simulink model "single_camera_xy_tracking_base_cv_kf_pre_fix"  (R2025b)
settings: Solver=FixedStepDiscrete  StartTime=0  StopTime=T_end  FixedStep=Ts  RelTol=1e-3
InitFcn:
  | config_dir=fullfile(fileparts(get_param(bdroot,'FileName')),'..','config');
  | addpath(config_dir);
  | init_single_camera_xy_tracking_base_cv_kf;
values from neighbouring files (symbols this model uses):
  Kpx = parameters(3)    [build_single_camera_joint_velocity_direct.m]    (also in build_single_camera_joint_velocity_direct1.m)
  Kpy = parameters(4);",  "k_ff=parameters(5)    [build_single_camera_joint_velocity_direct.m]    (also in build_single_camera_joint_velocity_direct1.m)
  Z_hat = parameters(2)    [build_single_camera_joint_velocity_direct.m]    (also in build_single_camera_joint_velocity_direct1.m)
undefined symbols (not defined in the file or in its folder): a_xy_max, controller_enable, data, data_SL_Info, ekf_reset_timeout_sec, enable_ekf_feedforward, enable_proportional, ff_ramp_time, joint_state_timeout_sec, k_ff, measurement_reset_timeout, nis_position_threshold, nis_velocity_threshold, P0, Q_kf, R_position, R_velocity, required_valid_frames, target_timeout_sec, Ts, v_xy_max
libraries: ros2lib x5, robotmaniplib x2
Description:
  | Base-frame four-state CV Kalman Filter. Python velocity is camera-frame relative velocity; measured camera twist is compensated before KF updates.
settings Model: Creator=ASUS  LastModifiedBy=ASUS
settings DataIOCC: SignalLogging=off

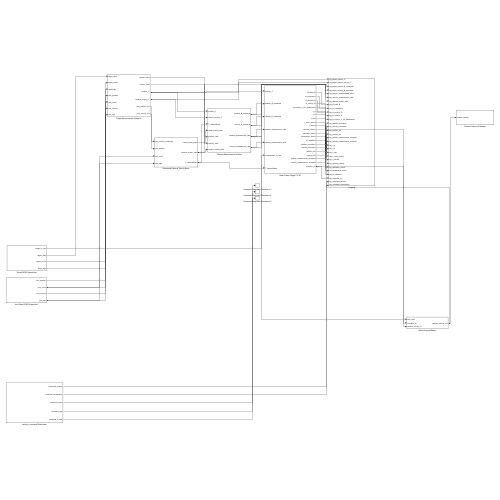
[thumbnail: Simulink's stored preview of the top-level diagram]
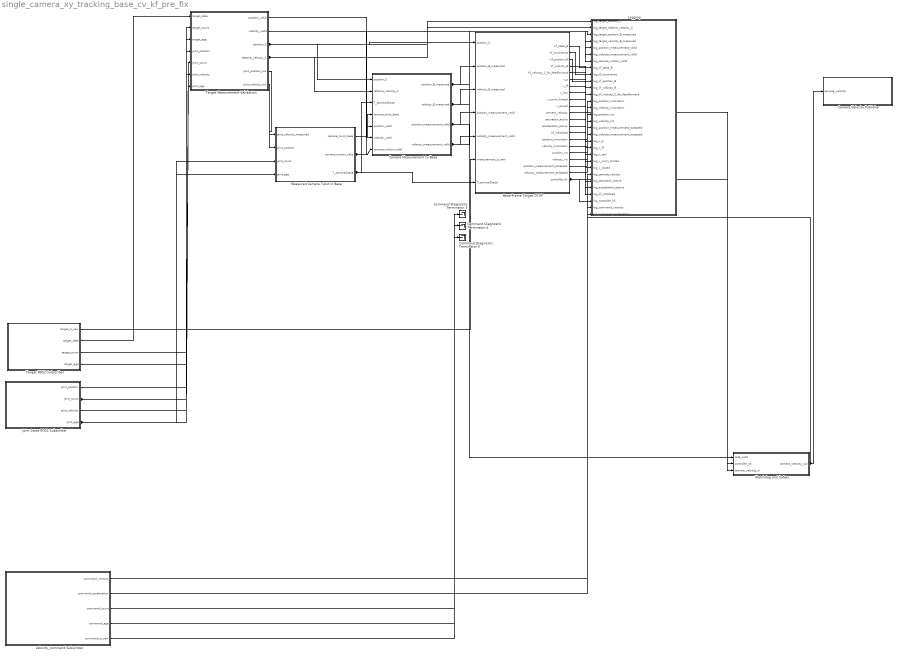
== system single_camera_xy_tracking_base_cv_kf_pre_fix ==
  Base-Frame Target CV KF : Subsystem
  Camera Measurement to Base : Subsystem
  Camera Velocity Publisher : Subsystem
  Command Diagnostic Terminator 3 : Terminator
  Command Diagnostic Terminator 4 : Terminator
  Command Diagnostic Terminator 5 : Terminator
  Joint State ROS2 Subscriber : Subsystem
  Logging : Subsystem
  Measured Camera Twist in Base : Subsystem
  Target Measurement Validation : Subsystem
  Target ROS2 Subscriber : Subsystem
  Watchdog and Safety : Subsystem
  velocity_command Subscriber : Subsystem
  wires:
  Target ROS2 Subscriber/2(target_data) -> Target Measurement Validation/1(target_data)
  Target ROS2 Subscriber/3(target_count) -> Target Measurement Validation/2(target_count)
  Target ROS2 Subscriber/4(target_age) -> Target Measurement Validation/3(target_age)
  Joint State ROS2 Subscriber/1(joint_position) -> Target Measurement Validation/4(joint_position)
  Joint State ROS2 Subscriber/2(joint_count) -> Target Measurement Validation/5(joint_count), Measured Camera Twist in Base/3(joint_count)
  Joint State ROS2 Subscriber/3(joint_velocity) -> Target Measurement Validation/6(joint_velocity)
  Joint State ROS2 Subscriber/4(joint_age) -> Target Measurement Validation/7(joint_age), Measured Camera Twist in Base/4(joint_age)
  Target Measurement Validation/6(joint_velocity_out) -> Measured Camera Twist in Base/1(joint_velocity_measured)
  Target Measurement Validation/5(joint_position_out) -> Measured Camera Twist in Base/2(joint_position)
  Target Measurement Validation/3(position_C) -> Camera Measurement to Base/1(position_C), Base-Frame Target CV KF/1(position_C), Logging/1(log_target_position_C)
  Target Measurement Validation/4(relative_velocity_C) -> Camera Measurement to Base/2(relative_velocity_C), Logging/2(log_target_relative_velocity_C)
  Measured Camera Twist in Base/3(T_camera2base) -> Camera Measurement to Base/3(T_camera2base), Base-Frame Target CV KF/7(T_camera2base)
  Measured Camera Twist in Base/1(camera_twist_base) -> Camera Measurement to Base/4(camera_twist_base)
  Target Measurement Validation/1(position_valid) -> Camera Measurement to Base/5(position_valid)
  Target Measurement Validation/2(velocity_valid) -> Camera Measurement to Base/6(velocity_valid)
  Measured Camera Twist in Base/2(camera_motion_valid) -> Camera Measurement to Base/7(camera_motion_valid), Logging/7(log_camera_motion_valid)
  Camera Measurement to Base/1(position_B_measured) -> Base-Frame Target CV KF/2(position_B_measured), Logging/3(log_target_position_B_measured)
  Camera Measurement to Base/2(velocity_B_measured) -> Base-Frame Target CV KF/3(velocity_B_measured), Logging/4(log_target_velocity_B_measured)
  Camera Measurement to Base/3(position_measurement_valid) -> Base-Frame Target CV KF/4(position_measurement_valid), Watchdog and Safety/1(safe_valid), Logging/5(log_position_measurement_valid)
  Camera Measurement to Base/4(velocity_measurement_valid) -> Base-Frame Target CV KF/5(velocity_measurement_valid), Logging/6(log_velocity_measurement_valid)
  Target ROS2 Subscriber/1(target_is_new) -> Base-Frame Target CV KF/6(measurement_is_new)
  Base-Frame Target CV KF/21(controller_ok) -> Watchdog and Safety/2(controller_ok), Logging/28(log_controller_ok)
  Base-Frame Target CV KF/11(camera_velocity) -> Watchdog and Safety/3(camera_velocity_in)
  Watchdog and Safety/1(camera_velocity_out) -> Camera Velocity Publisher/1(camera_velocity), Logging/24(log_camera_velocity)
  Base-Frame Target CV KF/1(kf_state_B) -> Logging/8(log_kf_state_B)
  Base-Frame Target CV KF/2(kf_covariance) -> Logging/9(log_kf_covariance)
  Base-Frame Target CV KF/3(kf_position_B) -> Logging/10(log_kf_position_B)
  Base-Frame Target CV KF/4(kf_velocity_B) -> Logging/11(log_kf_velocity_B)
  Base-Frame Target CV KF/5(kf_velocity_C_for_feedforward) -> Logging/12(log_kf_velocity_C_for_feedforward)
  Base-Frame Target CV KF/15(position_innovation) -> Logging/13(log_position_innovation)
  Base-Frame Target CV KF/16(velocity_innovation) -> Logging/14(log_velocity_innovation)
  Base-Frame Target CV KF/17(position_nis) -> Logging/15(log_position_nis)
  Base-Frame Target CV KF/18(velocity_nis) -> Logging/16(log_velocity_nis)
  Base-Frame Target CV KF/19(position_measurement_accepted) -> Logging/17(log_position_measurement_accepted)
  Base-Frame Target CV KF/20(velocity_measurement_accepted) -> Logging/18(log_velocity_measurement_accepted)
  Base-Frame Target CV KF/6(v_p) -> Logging/19(log_v_p)
  Base-Frame Target CV KF/7(v_ff) -> Logging/20(log_v_ff)
  Base-Frame Target CV KF/8(v_raw) -> Logging/21(log_v_raw)
  Base-Frame Target CV KF/9(v_norm_limited) -> Logging/22(log_v_norm_limited)
  Base-Frame Target CV KF/10(v_issued) -> Logging/23(log_v_issued)
  Base-Frame Target CV KF/12(saturation_active) -> Logging/25(log_saturation_active)
  Base-Frame Target CV KF/13(acceleration_active) -> Logging/26(log_acceleration_active)
  Base-Frame Target CV KF/14(kf_initialized) -> Logging/27(log_kf_initialized)
  velocity_command Subscriber/1(command_velocity) -> Logging/29(log_command_velocity)
  velocity_command Subscriber/2(command_acceleration) -> Logging/30(log_command_acceleration)
  velocity_command Subscriber/3(command_count) -> Command Diagnostic Terminator 3/1
  velocity_command Subscriber/4(command_age) -> Command Diagnostic Terminator 4/1
  velocity_command Subscriber/5(command_is_new) -> Command Diagnostic Terminator 5/1

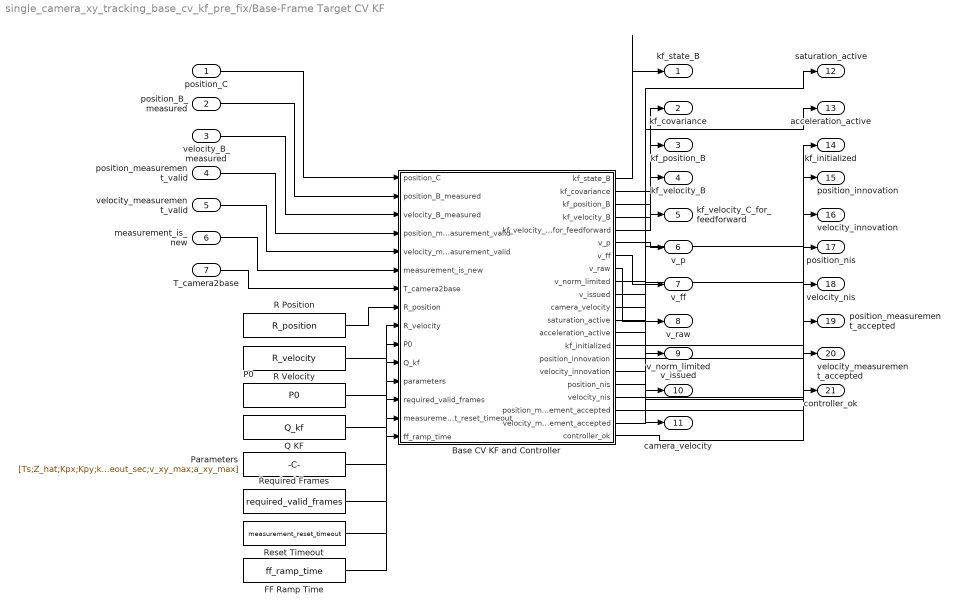
== system single_camera_xy_tracking_base_cv_kf_pre_fix/Base-Frame Target CV KF ==
  position_C : Inport
  position_B_measured : Inport  Port=2
  velocity_B_measured : Inport  Port=3
  position_measurement_valid : Inport  Port=4
  velocity_measurement_valid : Inport  Port=5
  measurement_is_new : Inport  Port=6
  T_camera2base : Inport  Port=7
  Base CV KF and Controller : MATLAB Function  TreatAsAtomicUnit=on
  FF Ramp Time : Constant  Value=ff_ramp_time
  P0 : Constant  Value=P0
  Parameters : Constant  Value=[Ts;Z_hat;Kpx;Kpy;k_ff;nis_position_threshold;nis_velocity_threshold;double(enable_proportional);double(enable_ekf_feedforward);double(controller_enable);ekf_reset_timeout_sec;v_xy_max;a_xy_max]
  Q KF : Constant  Value=Q_kf
  R Position : Constant  Value=R_position
  R Velocity : Constant  Value=R_velocity
  Required Frames : Constant  Value=required_valid_frames
  Reset Timeout : Constant  Value=measurement_reset_timeout
  kf_state_B : Outport
  kf_covariance : Outport  Port=2
  kf_position_B : Outport  Port=3
  kf_velocity_B : Outport  Port=4
  kf_velocity_C_for_feedforward : Outport  Port=5
  v_p : Outport  Port=6
  v_ff : Outport  Port=7
  v_raw : Outport  Port=8
  v_norm_limited : Outport  Port=9
  v_issued : Outport  Port=10
  camera_velocity : Outport  Port=11
  saturation_active : Outport  Port=12
  acceleration_active : Outport  Port=13
  kf_initialized : Outport  Port=14
  position_innovation : Outport  Port=15
  velocity_innovation : Outport  Port=16
  position_nis : Outport  Port=17
  velocity_nis : Outport  Port=18
  position_measurement_accepted : Outport  Port=19
  velocity_measurement_accepted : Outport  Port=20
  controller_ok : Outport  Port=21
  wires:
  position_C/1 -> Base CV KF and Controller/1(position_C)
  position_B_measured/1 -> Base CV KF and Controller/2(position_B_measured)
  velocity_B_measured/1 -> Base CV KF and Controller/3(velocity_B_measured)
  position_measurement_valid/1 -> Base CV KF and Controller/4(position_measurement_valid)
  velocity_measurement_valid/1 -> Base CV KF and Controller/5(velocity_measurement_valid)
  measurement_is_new/1 -> Base CV KF and Controller/6(measurement_is_new)
  T_camera2base/1 -> Base CV KF and Controller/7(T_camera2base)
  R Position/1 -> Base CV KF and Controller/8(R_position)
  R Velocity/1 -> Base CV KF and Controller/9(R_velocity)
  P0/1 -> Base CV KF and Controller/10(P0)
  Q KF/1 -> Base CV KF and Controller/11(Q_kf)
  Parameters/1 -> Base CV KF and Controller/12(parameters)
  Required Frames/1 -> Base CV KF and Controller/13(required_valid_frames)
  Reset Timeout/1 -> Base CV KF and Controller/14(measurement_reset_timeout)
  FF Ramp Time/1 -> Base CV KF and Controller/15(ff_ramp_time)
  Base CV KF and Controller/1(kf_state_B) -> kf_state_B/1
  Base CV KF and Controller/2(kf_covariance) -> kf_covariance/1
  Base CV KF and Controller/3(kf_position_B) -> kf_position_B/1
  Base CV KF and Controller/4(kf_velocity_B) -> kf_velocity_B/1
  Base CV KF and Controller/5(kf_velocity_C_for_feedforward) -> kf_velocity_C_for_feedforward/1
  Base CV KF and Controller/6(v_p) -> v_p/1
  Base CV KF and Controller/7(v_ff) -> v_ff/1
  Base CV KF and Controller/8(v_raw) -> v_raw/1
  Base CV KF and Controller/9(v_norm_limited) -> v_norm_limited/1
  Base CV KF and Controller/10(v_issued) -> v_issued/1
  Base CV KF and Controller/11(camera_velocity) -> camera_velocity/1
  Base CV KF and Controller/12(saturation_active) -> saturation_active/1
  Base CV KF and Controller/13(acceleration_active) -> acceleration_active/1
  Base CV KF and Controller/14(kf_initialized) -> kf_initialized/1
  Base CV KF and Controller/15(position_innovation) -> position_innovation/1
  Base CV KF and Controller/16(velocity_innovation) -> velocity_innovation/1
  Base CV KF and Controller/17(position_nis) -> position_nis/1
  Base CV KF and Controller/18(velocity_nis) -> velocity_nis/1
  Base CV KF and Controller/19(position_measurement_accepted) -> position_measurement_accepted/1
  Base CV KF and Controller/20(velocity_measurement_accepted) -> velocity_measurement_accepted/1
  Base CV KF and Controller/21(controller_ok) -> controller_ok/1

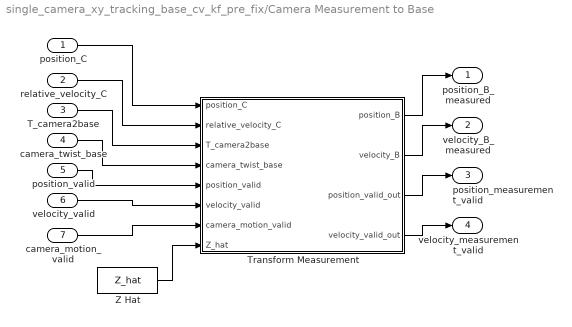
== system single_camera_xy_tracking_base_cv_kf_pre_fix/Camera Measurement to Base ==
  position_C : Inport
  relative_velocity_C : Inport  Port=2
  T_camera2base : Inport  Port=3
  camera_twist_base : Inport  Port=4
  position_valid : Inport  Port=5
  velocity_valid : Inport  Port=6
  camera_motion_valid : Inport  Port=7
  Transform Measurement : MATLAB Function  TreatAsAtomicUnit=on
  Z Hat : Constant  Value=Z_hat
  position_B_measured : Outport
  velocity_B_measured : Outport  Port=2
  position_measurement_valid : Outport  Port=3
  velocity_measurement_valid : Outport  Port=4
  wires:
  position_C/1 -> Transform Measurement/1(position_C)
  relative_velocity_C/1 -> Transform Measurement/2(relative_velocity_C)
  T_camera2base/1 -> Transform Measurement/3(T_camera2base)
  camera_twist_base/1 -> Transform Measurement/4(camera_twist_base)
  position_valid/1 -> Transform Measurement/5(position_valid)
  velocity_valid/1 -> Transform Measurement/6(velocity_valid)
  camera_motion_valid/1 -> Transform Measurement/7(camera_motion_valid)
  Z Hat/1 -> Transform Measurement/8(Z_hat)
  Transform Measurement/1(position_B) -> position_B_measured/1
  Transform Measurement/2(velocity_B) -> velocity_B_measured/1
  Transform Measurement/3(position_valid_out) -> position_measurement_valid/1
  Transform Measurement/4(velocity_valid_out) -> velocity_measurement_valid/1

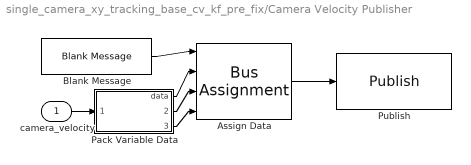
== system single_camera_xy_tracking_base_cv_kf_pre_fix/Camera Velocity Publisher ==
  camera_velocity : Inport
  Assign Data : BusAssignment  AssignedSignals=data,data_SL_Info.CurrentLength,data_SL_Info.ReceivedLength
  Blank Message : ros2lib/Blank Message  messageClass=Message  entityType=std_msgs/Float64MultiArray  messageType=std_msgs/Float64MultiArray  SampleTime=Ts
  Pack Variable Data : MATLAB Function  TreatAsAtomicUnit=on
  Publish : ros2lib/Publish  topicSource=Select from ROS network  topic=/simulink/camera_velocity  messageType=std_msgs/Float64MultiArray  QOSHistory=Keep last  QOSDepth=1  QOSReliability=Reliable  QOSDurability=Volatile  QOSDeadline=Inf  QOSLifespan=Inf  QOSLiveliness=Automatic  QOSLeaseDuration=Inf  QOSAvoidROSNamespaceConventions=off
  wires:
  Blank Message/1 -> Assign Data/1
  Assign Data/1 -> Publish/1
  camera_velocity/1 -> Pack Variable Data/1(camera_velocity)
  Pack Variable Data/1(data) -> Assign Data/2
  Pack Variable Data/2(current_length) -> Assign Data/3
  Pack Variable Data/3(received_length) -> Assign Data/4

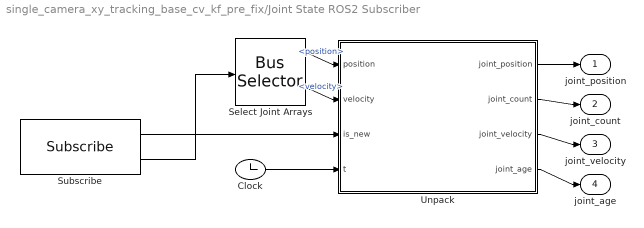
== system single_camera_xy_tracking_base_cv_kf_pre_fix/Joint State ROS2 Subscriber ==
  Clock : Clock
  Select Joint Arrays : BusSelector  OutputSignals=position,velocity
  Subscribe : ros2lib/Subscribe  topicSource=Select from ROS network  topic=/franka/joint_states  messageType=sensor_msgs/JointState  sampleTime=Ts  QOSHistory=Keep last  QOSDepth=1  QOSReliability=Best effort  QOSDurability=Volatile  QOSDeadline=Inf  QOSLifespan=Inf  QOSLiveliness=Automatic  QOSLeaseDuration=Inf  QOSAvoidROSNamespaceConventions=off
  Unpack : MATLAB Function  TreatAsAtomicUnit=on
  joint_position : Outport
  joint_count : Outport  Port=2
  joint_velocity : Outport  Port=3
  joint_age : Outport  Port=4
  wires:
  Unpack/1(joint_position) -> joint_position/1
  Unpack/2(joint_count) -> joint_count/1
  Unpack/3(joint_velocity) -> joint_velocity/1
  Unpack/4(joint_age) -> joint_age/1
  Select Joint Arrays/1 -> Unpack/1(position)  "<position>"
  Select Joint Arrays/2 -> Unpack/2(velocity)  "<velocity>"
  Clock/1 -> Unpack/4(t)
  Subscribe/2 -> Select Joint Arrays/1
  Subscribe/1 -> Unpack/3(is_new)

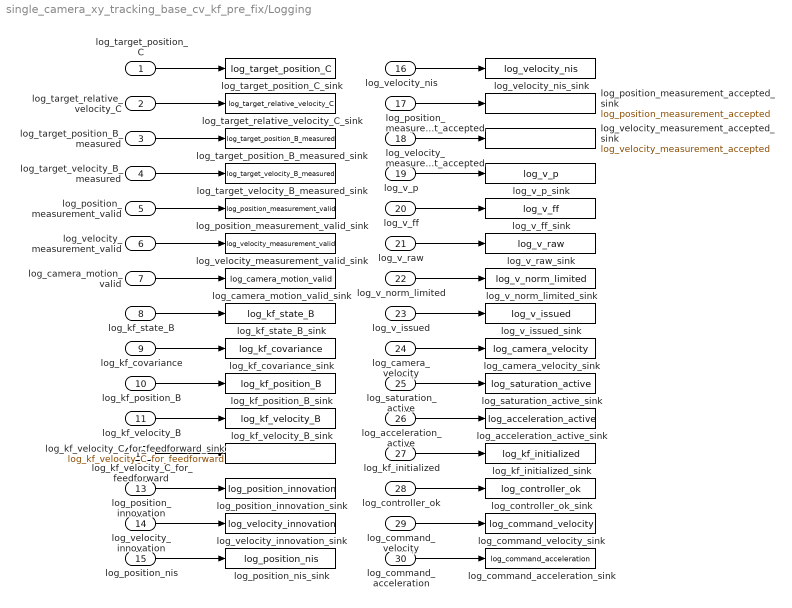
== system single_camera_xy_tracking_base_cv_kf_pre_fix/Logging ==
  log_target_position_C : Inport
  log_target_relative_velocity_C : Inport  Port=2
  log_target_position_B_measured : Inport  Port=3
  log_target_velocity_B_measured : Inport  Port=4
  log_position_measurement_valid : Inport  Port=5
  log_velocity_measurement_valid : Inport  Port=6
  log_camera_motion_valid : Inport  Port=7
  log_kf_state_B : Inport  Port=8
  log_kf_covariance : Inport  Port=9
  log_kf_position_B : Inport  Port=10
  log_kf_velocity_B : Inport  Port=11
  log_kf_velocity_C_for_feedforward : Inport  Port=12
  log_position_innovation : Inport  Port=13
  log_velocity_innovation : Inport  Port=14
  log_position_nis : Inport  Port=15
  log_velocity_nis : Inport  Port=16
  log_position_measurement_accepted : Inport  Port=17
  log_velocity_measurement_accepted : Inport  Port=18
  log_v_p : Inport  Port=19
  log_v_ff : Inport  Port=20
  log_v_raw : Inport  Port=21
  log_v_norm_limited : Inport  Port=22
  log_v_issued : Inport  Port=23
  log_camera_velocity : Inport  Port=24
  log_saturation_active : Inport  Port=25
  log_acceleration_active : Inport  Port=26
  log_kf_initialized : Inport  Port=27
  log_controller_ok : Inport  Port=28
  log_command_velocity : Inport  Port=29
  log_command_acceleration : Inport  Port=30
  log_acceleration_active_sink : ToWorkspace  VariableName=log_acceleration_active  SaveFormat=Timeseries  SampleTime=-1
  log_camera_motion_valid_sink : ToWorkspace  VariableName=log_camera_motion_valid  SaveFormat=Timeseries  SampleTime=-1
  log_camera_velocity_sink : ToWorkspace  VariableName=log_camera_velocity  SaveFormat=Timeseries  SampleTime=-1
  log_command_acceleration_sink : ToWorkspace  VariableName=log_command_acceleration  SaveFormat=Timeseries  SampleTime=-1
  log_command_velocity_sink : ToWorkspace  VariableName=log_command_velocity  SaveFormat=Timeseries  SampleTime=-1
  log_controller_ok_sink : ToWorkspace  VariableName=log_controller_ok  SaveFormat=Timeseries  SampleTime=-1
  log_kf_covariance_sink : ToWorkspace  VariableName=log_kf_covariance  SaveFormat=Timeseries  SampleTime=-1
  log_kf_initialized_sink : ToWorkspace  VariableName=log_kf_initialized  SaveFormat=Timeseries  SampleTime=-1
  log_kf_position_B_sink : ToWorkspace  VariableName=log_kf_position_B  SaveFormat=Timeseries  SampleTime=-1
  log_kf_state_B_sink : ToWorkspace  VariableName=log_kf_state_B  SaveFormat=Timeseries  SampleTime=-1
  log_kf_velocity_B_sink : ToWorkspace  VariableName=log_kf_velocity_B  SaveFormat=Timeseries  SampleTime=-1
  log_kf_velocity_C_for_feedforward_sink : ToWorkspace  VariableName=log_kf_velocity_C_for_feedforward  SaveFormat=Timeseries  SampleTime=-1
  log_position_innovation_sink : ToWorkspace  VariableName=log_position_innovation  SaveFormat=Timeseries  SampleTime=-1
  log_position_measurement_accepted_sink : ToWorkspace  VariableName=log_position_measurement_accepted  SaveFormat=Timeseries  SampleTime=-1
  log_position_measurement_valid_sink : ToWorkspace  VariableName=log_position_measurement_valid  SaveFormat=Timeseries  SampleTime=-1
  log_position_nis_sink : ToWorkspace  VariableName=log_position_nis  SaveFormat=Timeseries  SampleTime=-1
  log_saturation_active_sink : ToWorkspace  VariableName=log_saturation_active  SaveFormat=Timeseries  SampleTime=-1
  log_target_position_B_measured_sink : ToWorkspace  VariableName=log_target_position_B_measured  SaveFormat=Timeseries  SampleTime=-1
  log_target_position_C_sink : ToWorkspace  VariableName=log_target_position_C  SaveFormat=Timeseries  SampleTime=-1
  log_target_relative_velocity_C_sink : ToWorkspace  VariableName=log_target_relative_velocity_C  SaveFormat=Timeseries  SampleTime=-1
  log_target_velocity_B_measured_sink : ToWorkspace  VariableName=log_target_velocity_B_measured  SaveFormat=Timeseries  SampleTime=-1
  log_v_ff_sink : ToWorkspace  VariableName=log_v_ff  SaveFormat=Timeseries  SampleTime=-1
  log_v_issued_sink : ToWorkspace  VariableName=log_v_issued  SaveFormat=Timeseries  SampleTime=-1
  log_v_norm_limited_sink : ToWorkspace  VariableName=log_v_norm_limited  SaveFormat=Timeseries  SampleTime=-1
  log_v_p_sink : ToWorkspace  VariableName=log_v_p  SaveFormat=Timeseries  SampleTime=-1
  log_v_raw_sink : ToWorkspace  VariableName=log_v_raw  SaveFormat=Timeseries  SampleTime=-1
  log_velocity_innovation_sink : ToWorkspace  VariableName=log_velocity_innovation  SaveFormat=Timeseries  SampleTime=-1
  log_velocity_measurement_accepted_sink : ToWorkspace  VariableName=log_velocity_measurement_accepted  SaveFormat=Timeseries  SampleTime=-1
  log_velocity_measurement_valid_sink : ToWorkspace  VariableName=log_velocity_measurement_valid  SaveFormat=Timeseries  SampleTime=-1
  log_velocity_nis_sink : ToWorkspace  VariableName=log_velocity_nis  SaveFormat=Timeseries  SampleTime=-1
  wires:
  log_target_position_C/1 -> log_target_position_C_sink/1
  log_target_relative_velocity_C/1 -> log_target_relative_velocity_C_sink/1
  log_target_position_B_measured/1 -> log_target_position_B_measured_sink/1
  log_target_velocity_B_measured/1 -> log_target_velocity_B_measured_sink/1
  log_position_measurement_valid/1 -> log_position_measurement_valid_sink/1
  log_velocity_measurement_valid/1 -> log_velocity_measurement_valid_sink/1
  log_camera_motion_valid/1 -> log_camera_motion_valid_sink/1
  log_kf_state_B/1 -> log_kf_state_B_sink/1
  log_kf_covariance/1 -> log_kf_covariance_sink/1
  log_kf_position_B/1 -> log_kf_position_B_sink/1
  log_kf_velocity_B/1 -> log_kf_velocity_B_sink/1
  log_kf_velocity_C_for_feedforward/1 -> log_kf_velocity_C_for_feedforward_sink/1
  log_position_innovation/1 -> log_position_innovation_sink/1
  log_velocity_innovation/1 -> log_velocity_innovation_sink/1
  log_position_nis/1 -> log_position_nis_sink/1
  log_velocity_nis/1 -> log_velocity_nis_sink/1
  log_position_measurement_accepted/1 -> log_position_measurement_accepted_sink/1
  log_velocity_measurement_accepted/1 -> log_velocity_measurement_accepted_sink/1
  log_v_p/1 -> log_v_p_sink/1
  log_v_ff/1 -> log_v_ff_sink/1
  log_v_raw/1 -> log_v_raw_sink/1
  log_v_norm_limited/1 -> log_v_norm_limited_sink/1
  log_v_issued/1 -> log_v_issued_sink/1
  log_camera_velocity/1 -> log_camera_velocity_sink/1
  log_saturation_active/1 -> log_saturation_active_sink/1
  log_acceleration_active/1 -> log_acceleration_active_sink/1
  log_kf_initialized/1 -> log_kf_initialized_sink/1
  log_controller_ok/1 -> log_controller_ok_sink/1
  log_command_velocity/1 -> log_command_velocity_sink/1
  log_command_acceleration/1 -> log_command_acceleration_sink/1

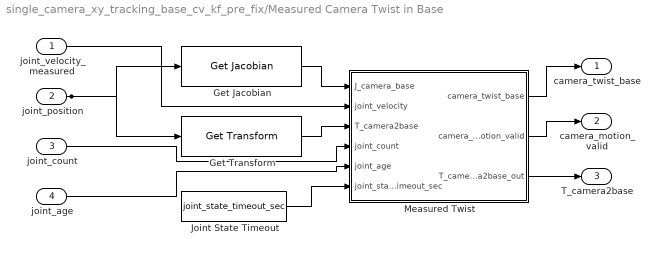
== system single_camera_xy_tracking_base_cv_kf_pre_fix/Measured Camera Twist in Base ==
  joint_velocity_measured : Inport
  joint_position : Inport  Port=2
  joint_count : Inport  Port=3
  joint_age : Inport  Port=4
  Get Jacobian : robotmaniplib/Get Jacobian  RigidBodyTree=fr3_camera_robot  EndEffector=camera_link  SimulateUsing=Interpreted execution
  Get Transform : robotmaniplib/Get Transform  RigidBodyTree=fr3_camera_robot  SourceBody=camera_link  TargetBody=base  SimulateUsing=Interpreted execution
  Joint State Timeout : Constant  Value=joint_state_timeout_sec
  Measured Twist : MATLAB Function  TreatAsAtomicUnit=on
  camera_twist_base : Outport
  camera_motion_valid : Outport  Port=2
  T_camera2base : Outport  Port=3
  wires:
  joint_position/1 -> Get Jacobian/1, Get Transform/1
  Get Jacobian/1 -> Measured Twist/1(J_camera_base)
  joint_velocity_measured/1 -> Measured Twist/2(joint_velocity)
  Get Transform/1 -> Measured Twist/3(T_camera2base)
  joint_count/1 -> Measured Twist/4(joint_count)
  joint_age/1 -> Measured Twist/5(joint_age)
  Joint State Timeout/1 -> Measured Twist/6(joint_state_timeout_sec)
  Measured Twist/1(camera_twist_base) -> camera_twist_base/1
  Measured Twist/2(camera_motion_valid) -> camera_motion_valid/1
  Measured Twist/3(T_camera2base_out) -> T_camera2base/1

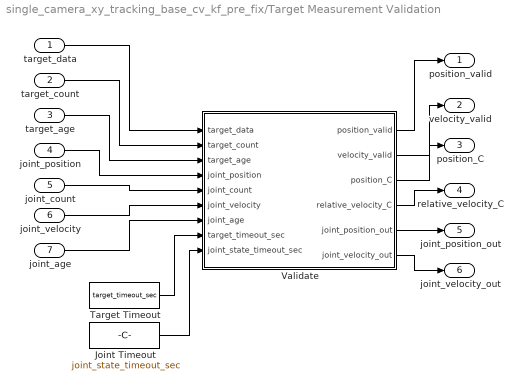
== system single_camera_xy_tracking_base_cv_kf_pre_fix/Target Measurement Validation ==
  target_data : Inport
  target_count : Inport  Port=2
  target_age : Inport  Port=3
  joint_position : Inport  Port=4
  joint_count : Inport  Port=5
  joint_velocity : Inport  Port=6
  joint_age : Inport  Port=7
  Joint Timeout : Constant  Value=joint_state_timeout_sec
  Target Timeout : Constant  Value=target_timeout_sec
  Validate : MATLAB Function  TreatAsAtomicUnit=on
  position_valid : Outport
  velocity_valid : Outport  Port=2
  position_C : Outport  Port=3
  relative_velocity_C : Outport  Port=4
  joint_position_out : Outport  Port=5
  joint_velocity_out : Outport  Port=6
  wires:
  target_data/1 -> Validate/1(target_data)
  target_count/1 -> Validate/2(target_count)
  target_age/1 -> Validate/3(target_age)
  joint_position/1 -> Validate/4(joint_position)
  joint_count/1 -> Validate/5(joint_count)
  joint_velocity/1 -> Validate/6(joint_velocity)
  joint_age/1 -> Validate/7(joint_age)
  Target Timeout/1 -> Validate/8(target_timeout_sec)
  Joint Timeout/1 -> Validate/9(joint_state_timeout_sec)
  Validate/1(position_valid) -> position_valid/1
  Validate/2(velocity_valid) -> velocity_valid/1
  Validate/3(position_C) -> position_C/1
  Validate/4(relative_velocity_C) -> relative_velocity_C/1
  Validate/5(joint_position_out) -> joint_position_out/1
  Validate/6(joint_velocity_out) -> joint_velocity_out/1

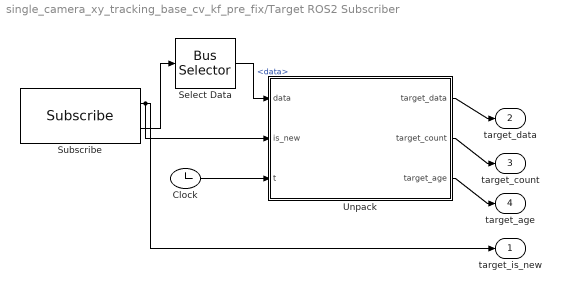
== system single_camera_xy_tracking_base_cv_kf_pre_fix/Target ROS2 Subscriber ==
  Clock : Clock
  Select Data : BusSelector  OutputSignals=data
  Subscribe : ros2lib/Subscribe  topicSource=Select from ROS network  topic=/apriltag_detector/target_position  messageType=std_msgs/Float64MultiArray  sampleTime=Ts  QOSHistory=Keep last  QOSDepth=1  QOSReliability=Best effort  QOSDurability=Volatile  QOSDeadline=Inf  QOSLifespan=Inf  QOSLiveliness=Automatic  QOSLeaseDuration=Inf  QOSAvoidROSNamespaceConventions=off
  Unpack : MATLAB Function  TreatAsAtomicUnit=on
  target_is_new : Outport
  target_data : Outport  Port=2
  target_count : Outport  Port=3
  target_age : Outport  Port=4
  wires:
  Unpack/1(target_data) -> target_data/1
  Unpack/2(target_count) -> target_count/1
  Unpack/3(target_age) -> target_age/1
  Select Data/1 -> Unpack/1(data)  "<data>"
  Clock/1 -> Unpack/3(t)
  Subscribe/2 -> Select Data/1
  Subscribe/1 -> Unpack/2(is_new), target_is_new/1

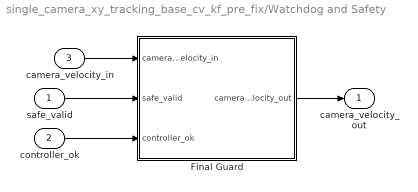
== system single_camera_xy_tracking_base_cv_kf_pre_fix/Watchdog and Safety ==
  safe_valid : Inport
  controller_ok : Inport  Port=2
  camera_velocity_in : Inport  Port=3
  Final Guard : MATLAB Function  TreatAsAtomicUnit=on
  camera_velocity_out : Outport
  wires:
  camera_velocity_in/1 -> Final Guard/1(camera_velocity_in)
  safe_valid/1 -> Final Guard/2(safe_valid)
  controller_ok/1 -> Final Guard/3(controller_ok)
  Final Guard/1(camera_velocity_out) -> camera_velocity_out/1

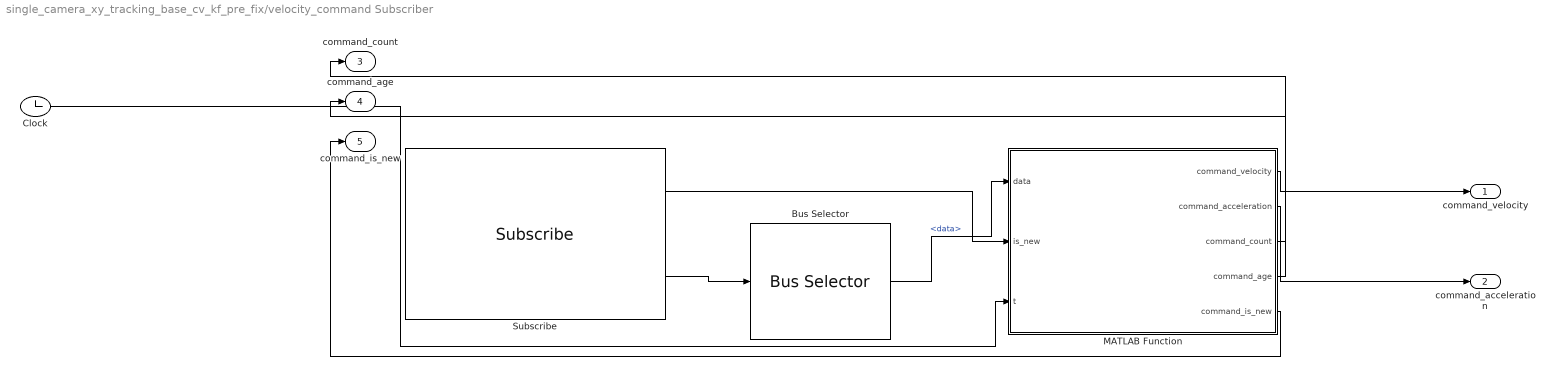
== system single_camera_xy_tracking_base_cv_kf_pre_fix/velocity_command Subscriber ==
  Bus Selector : BusSelector  OutputSignals=data
  Clock : Clock
  MATLAB Function : MATLAB Function  TreatAsAtomicUnit=on
  Subscribe : ros2lib/Subscribe  topicSource=Specify your own  topic=/joint_velocity_example_controller/commands  messageType=std_msgs/Float64MultiArray  sampleTime=-1  QOSHistory=Keep last  QOSDepth=10  QOSReliability=Reliable  QOSDurability=Volatile  QOSDeadline=Inf  QOSLifespan=Inf  QOSLiveliness=Automatic  QOSLeaseDuration=Inf  QOSAvoidROSNamespaceConventions=off
  command_velocity : Outport
  command_acceleration : Outport  Port=2
  command_count : Outport  Port=3
  command_age : Outport  Port=4
  command_is_new : Outport  Port=5
  wires:
  Subscribe/2 -> Bus Selector/1
  Bus Selector/1 -> MATLAB Function/1(data)  "<data>"
  MATLAB Function/2(command_acceleration) -> command_acceleration/1
  MATLAB Function/1(command_velocity) -> command_velocity/1
  Subscribe/1 -> MATLAB Function/2(is_new)
  Clock/1 -> MATLAB Function/3(t)
  MATLAB Function/3(command_count) -> command_count/1
  MATLAB Function/4(command_age) -> command_age/1
  MATLAB Function/5(command_is_new) -> command_is_new/1

== matlab function single_camera_xy_tracking_base_cv_kf_pre_fix/Base-Frame Target CV KF/Base CV KF and Controller ==
  data: position_C input size=[2 1]; kf_state_B output size=[4 1]; position_B_measured input size=[2 1]; velocity_B_measured input size=[2 1]; position_measurement_valid input; velocity_measurement_valid input; measurement_is_new input; T_camera2base input size=[4 4]; R_position input size=[2 2]; R_velocity input size=[2 2]; P0 input size=[4 4]; Q_kf input size=[4 4]; parameters input size=[13 1]; required_valid_frames input; measurement_reset_timeout input; ff_ramp_time input; kf_covariance output size=[4 4]; kf_position_B output size=[2 1]; kf_velocity_B output size=[2 1]; kf_velocity_C_for_feedforward output size=[2 1]; v_p output size=[2 1]; v_ff output size=[2 1]; v_raw output size=[2 1]; v_norm_limited output size=[2 1]; v_issued output size=[2 1]; camera_velocity output size=[6 1]; saturation_active output; acceleration_active output; kf_initialized output; position_innovation output size=[2 1]; velocity_innovation output size=[2 1]; position_nis output; velocity_nis output; position_measurement_accepted output; velocity_measurement_accepted output; controller_ok output
function [kf_state_B,kf_covariance,kf_position_B,kf_velocity_B, ...
    kf_velocity_C_for_feedforward,v_p,v_ff,v_raw,v_norm_limited,v_issued, ...
    camera_velocity,saturation_active,acceleration_active,kf_initialized, ...
    position_innovation,velocity_innovation,position_nis,velocity_nis, ...
    position_measurement_accepted,velocity_measurement_accepted,controller_ok] = ...
    fcn(position_C,position_B_measured,velocity_B_measured, ...
    position_measurement_valid,velocity_measurement_valid,measurement_is_new, ...
    T_camera2base,R_position,R_velocity,P0,Q_kf,parameters, ...
    required_valid_frames,measurement_reset_timeout,ff_ramp_time)
%#codegen
% Base 系四状态匀速 KF 与 P+KF 速度前馈控制器。
% 状态为 [X_B;Y_B;V_tx,B;V_ty,B]；预测严格为 x^-=A*x，不含相机速度 B 输入。
persistent x P position_C_hold elapsed initialized v_previous valid_streak kf_ready ff_ramp
if isempty(initialized)
    x=zeros(4,1); P=P0; position_C_hold=zeros(2,1); elapsed=0;
    initialized=false; v_previous=zeros(2,1); valid_streak=0;
    kf_ready=false; ff_ramp=0;
end

kf_state_B=x; kf_covariance=P; kf_position_B=x(1:2); kf_velocity_B=zeros(2,1);
kf_velocity_C_for_feedforward=zeros(2,1); v_p=zeros(2,1); v_ff=zeros(2,1);
v_raw=zeros(2,1); v_norm_limited=zeros(2,1); v_issued=zeros(2,1);
camera_velocity=zeros(6,1); saturation_active=false; acceleration_active=false;
kf_initialized=initialized&&kf_ready; position_innovation=zeros(2,1);
velocity_innovation=zeros(2,1); position_nis=NaN; velocity_nis=NaN;
position_measurement_accepted=false; velocity_measurement_accepted=false;
controller_ok=false;

if numel(parameters)<13, return; end
Ts=parameters(1); Z_hat=parameters(2); Kp=parameters(3:4); k_ff=parameters(5);
position_gate=parameters(6); velocity_gate=parameters(7);
enable_p=parameters(8)>.5; enable_ff=parameters(9)>.5;
controller_enable=parameters(10)>.5; v_xy_max=parameters(12); a_xy_max=parameters(13);
required_valid_frames=max(1,floor(required_valid_frames));
parameter_ok=all(isfinite(parameters(:))) && Ts>0 && Z_hat>0 && ...
    position_gate>0 && velocity_gate>0 && v_xy_max>0 && a_xy_max>0 && ...
    measurement_reset_timeout>=Ts && ff_ramp_time>0 && ...
    isequal(size(P0),[4 4]) && isequal(size(Q_kf),[4 4]) && ...
    isequal(size(R_position),[2 2]) && isequal(size(R_velocity),[2 2]) && ...
    all(isfinite([P0(:);Q_kf(:);R_position(:);R_velocity(:)]));
if ~parameter_ok
    x(:)=0; P=P0; position_C_hold(:)=0; elapsed=0; initialized=false;
    v_previous(:)=0; valid_streak=0; kf_ready=false; ff_ramp=0; return
end

A=[1 0 Ts 0;0 1 0 Ts;0 0 1 0;0 0 0 1];
new_position=position_measurement_valid>.5 && measurement_is_new>.5 && ...
    numel(position_B_measured)==2 && all(isfinite(position_B_measured(:)));
new_velocity=new_position && velocity_measurement_valid>.5 && ...
    numel(velocity_B_measured)==2 && all(isfinite(velocity_B_measured(:)));

if ~initialized
    if new_position
        x=[reshape(position_B_measured,2,1);zeros(2,1)];
        if new_velocity
            x(3:4)=reshape(velocity_B_measured,2,1);
            velocity_measurement_accepted=true;
        end
        P=P0; initialized=true; position_measurement_accepted=true;
    end
else
    [x,P,position_innovation,velocity_innovation,position_nis,velocity_nis, ...
        position_measurement_accepted,velocity_measurement_accepted]= ...
        base_cv_kf_step(x,P,position_B_measured,velocity_B_measured, ...
        new_position,new_velocity,A,Q_kf,R_position,R_velocity, ...
        position_gate,velocity_gate);
end

current_visual_valid=position_measurement_valid>.5 && ...
    numel(position_C)==2 && all(isfinite(position_C(:)));
if current_visual_valid&&measurement_is_new>.5
    position_C_hold=reshape(position_C,2,1);
end
if position_measurement_accepted
    elapsed=0; valid_streak=min(valid_streak+1,required_valid_frames);
    if valid_streak>=required_valid_frames, kf_ready=true; end
else
    elapsed=elapsed+Ts;
end

state_ok=all(isfinite(x)) && all(isfinite(P(:))) && all(diag(P)>=0) && ...
    norm(P-P','fro')<1e-6;
if elapsed>=measurement_reset_timeout || ~state_ok
    x(:)=0; P=P0; position_C_hold(:)=0; elapsed=0; initialized=false;
    v_previous(:)=0; valid_streak=0; kf_ready=false; ff_ramp=0;
    kf_state_B=x; kf_covariance=P; kf_position_B=x(1:2); return
end

kf_state_B=x; kf_covariance=P; kf_position_B=x(1:2);
if kf_ready, kf_velocity_B=x(3:4); end
kf_initialized=initialized&&kf_ready;
transform_ok=isequal(size(T_camera2base),[4 4]) && all(isfinite(T_camera2base(:)));
if transform_ok&&kf_ready
    velocity_C=T_camera2base(1:3,1:3)'*[x(3:4);0];
    if all(isfinite(velocity_C)), kf_velocity_C_for_feedforward=velocity_C(1:2); end
end

if ~current_visual_valid
    v_previous(:)=0; ff_ramp=0; return
end
if ~controller_enable||~initialized
    v_previous(:)=0; ff_ramp=0; return
end

% 与旧模型 Z_hat*Kp.*e 等价，保持相机系比例反馈的原符号约定。
if enable_p, v_p=Kp.*position_C_hold; end
% 前馈唯一来源：KF Base 系估计速度旋转回相机系后的 XY 分量。
if enable_ff&&kf_ready&&transform_ok
    ff_ramp=min(1,ff_ramp+Ts/ff_ramp_time);
    v_ff=ff_ramp*k_ff*kf_velocity_C_for_feedforward;
else
    ff_ramp=0;
end
v_raw=v_p+v_ff;
raw_norm=norm(v_raw); saturation_active=raw_norm>v_xy_max;
if saturation_active, v_norm_limited=v_raw*(v_xy_max/raw_norm); else, v_norm_limited=v_raw; end
delta=v_norm_limited-v_previous; delta_norm=norm(delta); delta_max=a_xy_max*Ts;
acceleration_active=delta_norm>delta_max;
if acceleration_active
    v_issued=v_previous+delta*(delta_max/delta_norm);
else
    v_issued=v_norm_limited;
end
controller_ok=all(isfinite([v_p;v_ff;v_raw;v_norm_limited;v_issued]));
if controller_ok
    v_previous=v_issued;
    camera_velocity=[v_issued;0;0;0;0];
else
    v_p(:)=0; v_ff(:)=0; v_raw(:)=0; v_norm_limited(:)=0; v_issued(:)=0;
    camera_velocity(:)=0; v_previous(:)=0; ff_ramp=0;
end
end

== matlab function single_camera_xy_tracking_base_cv_kf_pre_fix/Watchdog and Safety/Final Guard ==
  data: camera_velocity_in input size=[6 1]; camera_velocity_out output size=[6 1]; safe_valid input size=1; controller_ok input size=1
function camera_velocity_out = fcn(camera_velocity_in,safe_valid,controller_ok)
%#codegen
camera_velocity_out=zeros(6,1);
if safe_valid && controller_ok && all(isfinite(camera_velocity_in(:)))
    camera_velocity_out=camera_velocity_in;
    camera_velocity_out(3:6)=0;
end
end

== matlab function single_camera_xy_tracking_base_cv_kf_pre_fix/Camera Velocity Publisher/Pack Variable Data ==
  data: camera_velocity input size=[6 1]; data output size=[128 1]; current_length output size=1; received_length output size=1
function [data,current_length,received_length] = fcn(camera_velocity)
%#codegen
data=zeros(128,1); data(1:6)=camera_velocity;
current_length=uint32(6); received_length=uint32(6);
end

== matlab function single_camera_xy_tracking_base_cv_kf_pre_fix/velocity_command Subscriber/MATLAB Function ==
  data: data input; is_new input size=1; command_velocity output size=[7 1]; command_acceleration output size=[7 1]; t input size=1; command_count output size=1; command_age output size=1; command_is_new output size=1
function [command_velocity,command_acceleration,command_count, ...
    command_age,command_is_new]=fcn(data,is_new,t)
%#codegen
% 缓存最近一次合法的7关节命令速度，并输出消息年龄和新鲜度。
persistent last_velocity last_time last_count previous_velocity initialized
if isempty(initialized)
    last_velocity=zeros(7,1); previous_velocity=zeros(7,1);
    last_time=-1e6; last_count=0; initialized=false;
end
command_velocity=last_velocity; command_acceleration=zeros(7,1);
command_count=last_count; command_age=max(0,t-last_time);
command_is_new=false;
if ~is_new || numel(data)<7, return; end

current=zeros(7,1); valid=true;
for k=1:7
    current(k)=double(data(k)); valid=valid&&isfinite(current(k));
end
if ~valid, return; end
if initialized, command_acceleration=(current-previous_velocity)*120; end
last_velocity=current; previous_velocity=current; last_time=t;
last_count=7; initialized=true;
command_velocity=current; command_count=7; command_age=0;
command_is_new=true;
end

== matlab function single_camera_xy_tracking_base_cv_kf_pre_fix/Target ROS2 Subscriber/Unpack ==
  data: data input; target_data output size=[6 1]; is_new input size=1; t input size=1; target_count output size=1; target_age output size=1
function [target_data,target_count,target_age] = fcn(data,is_new,t)
%#codegen
% 缓存固定六元素消息：[valid,velocity_valid,X_C,Y_C,vx_rel_C,vy_rel_C]。
persistent last_data last_count last_time
if isempty(last_count)
    last_data=zeros(6,1); last_count=0; last_time=-1e6;
end
if is_new
    n=numel(data); last_data=zeros(6,1);
    for k=1:min(n,6), last_data(k)=double(data(k)); end
    last_count=double(n); last_time=t;
end
target_data=last_data;
target_count=last_count;
target_age=max(0,t-last_time);
end

== matlab function single_camera_xy_tracking_base_cv_kf_pre_fix/Target Measurement Validation/Validate ==
  data: target_data input size=[6 1]; position_valid output; target_count input; target_age input; joint_position input size=[7 1]; joint_count input; joint_velocity input size=[7 1]; joint_age input; target_timeout_sec input; joint_state_timeout_sec input; velocity_valid output; position_C output size=[2 1]; relative_velocity_C output size=[2 1]; joint_position_out output size=[7 1]; joint_velocity_out output size=[7 1]
function [position_valid,velocity_valid,position_C,relative_velocity_C, ...
    joint_position_out,joint_velocity_out] = fcn(target_data,target_count, ...
    target_age,joint_position,joint_count,joint_velocity,joint_age, ...
    target_timeout_sec,joint_state_timeout_sec)
%#codegen
% 校验视觉六元素载荷；末两项仅作为相机系目标—相机相对速度（m/s）。
[target_position_valid,target_velocity_valid,position_C,relative_velocity_C]= ...
    parse_target_measurement(target_data,target_count,target_age,target_timeout_sec);
joint_position_out=zeros(7,1);
joint_velocity_out=zeros(7,1);
geometry_ok=joint_count>=7 && numel(joint_position)>=7 && ...
    all(isfinite(joint_position(:)));
motion_ok=geometry_ok && numel(joint_velocity)>=7 && ...
    all(isfinite(joint_velocity(:))) && isfinite(joint_age) && ...
    joint_age>=0 && joint_age<=joint_state_timeout_sec;
if geometry_ok, joint_position_out=reshape(joint_position(1:7),7,1); end
if motion_ok, joint_velocity_out=reshape(joint_velocity(1:7),7,1); end
position_valid=target_position_valid&&geometry_ok;
velocity_valid=target_velocity_valid;
end

== matlab function single_camera_xy_tracking_base_cv_kf_pre_fix/Joint State ROS2 Subscriber/Unpack ==
  data: position input; joint_position output size=[7 1]; velocity input; is_new input size=1; t input size=1; joint_count output size=1; joint_velocity output size=[7 1]; joint_age output size=1
function [joint_position,joint_count,joint_velocity,joint_age] = fcn(position,velocity,is_new,t)
%#codegen
persistent last_q last_dq last_count last_time
if isempty(last_count), last_q=zeros(7,1); last_dq=zeros(7,1); last_count=0.0; last_time=-1.0e6; end
if is_new
    np=numel(position); nv=numel(velocity); last_q=zeros(7,1); last_dq=zeros(7,1);
    for k=1:min(np,7), last_q(k)=position(k); end
    for k=1:min(nv,7), last_dq(k)=velocity(k); end
    last_count=double(min(np,nv)); last_time=t;
end
joint_position=last_q; joint_count=last_count; joint_velocity=last_dq; joint_age=max(0.0,t-last_time);
end

== matlab function single_camera_xy_tracking_base_cv_kf_pre_fix/Measured Camera Twist in Base/Measured Twist ==
  data: J_camera_base input size=[6 7]; camera_twist_base output size=[6 1]; joint_velocity input size=[7 1]; T_camera2base input size=[4 4]; joint_count input; joint_age input; joint_state_timeout_sec input; camera_motion_valid output; T_camera2base_out output size=[4 4]
function [camera_twist_base,camera_motion_valid,T_camera2base_out] = fcn( ...
    J_camera_base,joint_velocity,T_camera2base,joint_count,joint_age, ...
    joint_state_timeout_sec)
%#codegen
% 用实测关节速度计算相机 Twist；geometricJacobian 顺序为 [omega_B;v_B]。
camera_twist_base=zeros(6,1);
T_camera2base_out=T_camera2base;
camera_motion_valid=false;
valid=isequal(size(J_camera_base),[6 7]) && all(isfinite(J_camera_base(:))) && ...
    numel(joint_velocity)>=7 && all(isfinite(joint_velocity(1:7))) && ...
    isequal(size(T_camera2base),[4 4]) && all(isfinite(T_camera2base(:))) && ...
    joint_count>=7 && isfinite(joint_age) && joint_age>=0 && ...
    joint_age<=joint_state_timeout_sec;
if ~valid, return; end
camera_twist_base=J_camera_base*reshape(joint_velocity(1:7),7,1);
camera_motion_valid=all(isfinite(camera_twist_base));
if ~camera_motion_valid, camera_twist_base(:)=0; end
end

== matlab function single_camera_xy_tracking_base_cv_kf_pre_fix/Camera Measurement to Base/Transform Measurement ==
  data: position_C input size=[2 1]; position_B output size=[2 1]; relative_velocity_C input size=[2 1]; T_camera2base input size=[4 4]; camera_twist_base input size=[6 1]; position_valid input; velocity_valid input; camera_motion_valid input; Z_hat input; velocity_B output size=[2 1]; position_valid_out output; velocity_valid_out output
function [position_B,velocity_B,position_valid_out,velocity_valid_out] = fcn( ...
    position_C,relative_velocity_C,T_camera2base,camera_twist_base, ...
    position_valid,velocity_valid,camera_motion_valid,Z_hat)
%#codegen
% 将相机系位置/相对速度转换为 Base 系位置/绝对速度，包含完整角速度补偿。
[position_B,velocity_B,position_valid_out,velocity_valid_out]= ...
    camera_measurement_to_base(position_C,relative_velocity_C,Z_hat, ...
    T_camera2base,camera_twist_base,position_valid,velocity_valid, ...
    camera_motion_valid);
end
